simulink model "Simulink_StateSpaceModel"  (R2014b)
settings: Solver=ode45  StartTime=0.0  StopTime=10.0  RelTol=1e-3
undefined symbols (not defined in the file): model
libraries: simulink x2
settings Model: Creator=rssalex  LastModifiedBy=rssalex

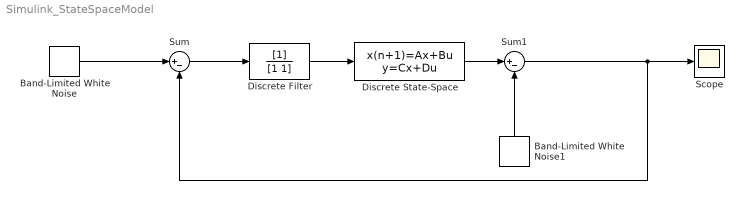
== system Simulink_StateSpaceModel ==
  Band-Limited White Noise : simulink/Sources/Band-Limited White Noise  Cov=[0.1]  Ts=0.2  seed=[101]
  Band-Limited White Noise1 : simulink/Sources/Band-Limited White Noise  Cov=[0.1]  Ts=0.2  seed=[101]
  Discrete Filter : DiscreteFilter  Denominator=[1 1]
  Discrete State-Space : DiscreteStateSpace  A=model.A  B=model.B  C=model.C  D=model.D
  Scope : Scope
  Sum : Sum  Inputs=|+-
  Sum1 : Sum  Inputs=|+-
  wires:
  Discrete Filter/1 -> Discrete State-Space/1
  Sum/1 -> Discrete Filter/1
  Band-Limited White Noise/1 -> Sum/1
  Discrete State-Space/1 -> Sum1/1
  Band-Limited White Noise1/1 -> Sum1/2
  Sum1/1 -> Sum/2, Scope/1
